simulink model "linCartPendulumEst"  (R2020a)
settings: Solver=VariableStepAuto  StartTime=0.0  StopTime=10.0  RelTol=1e-3
values from neighbouring files (symbols this model uses):
  xinit = [0;0;0;0]    [setupModelParameters.m]
undefined symbols (not defined in the file or in its folder): A, Ahat, B, Bhat, C, Chat, Dhat, xhatinit
settings Model: Creator=jamess  LastModifiedBy=jamessaunderson
settings DataIOCC: ReturnWorkspaceOutputs=off
settings DebuggingCC: ArithmeticOperatorsInVariantConditions=warning
settings SFSimCC: SimUseLocalCustomCode=off  CustomCodeUndefinedFunction=UseInterfaceOnly
settings RTWCC: RTWUseLocalCustomCode=off
settings CodeAppCC: StateflowObjectComments=on

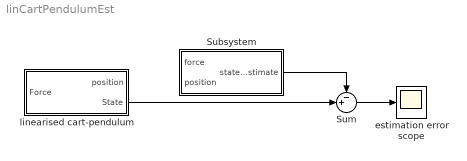
== system linCartPendulumEst ==
  Subsystem : Subsystem
  Sum : Sum  Inputs=-+|
  estimation error scope : Scope
  linearised cart-pendulum : Subsystem
  wires:
  Subsystem/1(state estimate) -> Sum/1
  linearised cart-pendulum/2(State) -> Sum/2
  Sum/1 -> estimation error scope/1

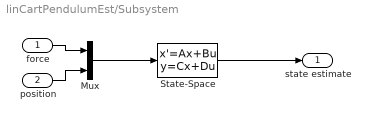
== system linCartPendulumEst/Subsystem ==
  force : Inport
  position : Inport  Port=2
  Mux : Mux  Inputs=2
  State-Space : StateSpace  A=Ahat  B=Bhat  C=Chat  D=Dhat  InitialCondition=xhatinit
  state estimate : Outport
  wires:
  State-Space/1 -> state estimate/1
  force/1 -> Mux/1
  position/1 -> Mux/2
  Mux/1 -> State-Space/1

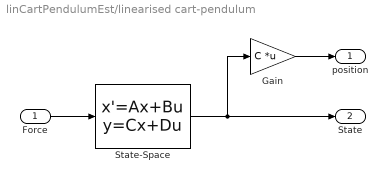
== system linCartPendulumEst/linearised cart-pendulum ==
  Force : Inport
  Gain : Gain  Gain=C  Multiplication=Matrix(K*u) (u vector)
  State-Space : StateSpace  A=A  B=B  C=eye(4)  D=zeros(4,1)  InitialCondition=xinit
  position : Outport
  State : Outport  Port=2
  wires:
  Force/1 -> State-Space/1
  State-Space/1 -> Gain/1, State/1
  Gain/1 -> position/1
